simulink model "HANcoder_E407_TTA_Chris"  (R2022b)
settings: Solver=FixedStepDiscrete  StartTime=0.0  StopTime=1  FixedStep=0.01  RelTol=1e-3
PreLoadFcn:
  | librarySetup
  | eval([bdroot,'_startup']) %Calling [modelName]_startup.m
values from neighbouring files (symbols this model uses):
  ClockOn = Simulink.Parameter    [HANcoder_E407_TTA_Chris_startup.m]    (also in HANcoder_E407_TTA_CombineModel_Membership_2022a_startup.m; HANcoder_E407_TTA_CombineModel_Membership_startup.m; HANcoder_E407_TTA_CombineModel_V2_startup.m; HANcoder_E407_TTA_CombineModel_startup.m)
  frequency_IRQ = 1000    [HANcoder_E407_TTA_Chris_startup.m]    (also in HANcoder_E407_TTA_CombineModel_Membership_2022a_startup.m; HANcoder_E407_TTA_CombineModel_Membership_startup.m; HANcoder_E407_TTA_CombineModel_V2_startup.m; HANcoder_E407_TTA_CombineModel_startup.m)
  idA = 4    [HANcoder_E407_TTA_Chris_startup.m]    (also in HANcoder_E407_TTA_CombineModel_Membership_2022a_startup.m; HANcoder_E407_TTA_CombineModel_Membership_startup.m; HANcoder_E407_TTA_CombineModel_V2_startup.m; HANcoder_E407_TTA_CombineModel_startup.m)
  idB = 6    [HANcoder_E407_TTA_Chris_startup.m]    (also in HANcoder_E407_TTA_CombineModel_Membership_2022a_startup.m; HANcoder_E407_TTA_CombineModel_Membership_startup.m; HANcoder_E407_TTA_CombineModel_V2_startup.m; HANcoder_E407_TTA_CombineModel_startup.m)
  matrixRows = Simulink.Parameter    [HANcoder_E407_TTA_Chris_startup.m]    (also in HANcoder_E407_TTA_CombineModel_Membership_2022a_startup.m; HANcoder_E407_TTA_CombineModel_Membership_startup.m; HANcoder_E407_TTA_CombineModel_V2_startup.m; HANcoder_E407_TTA_CombineModel_startup.m)
  MMBS1_ID = Simulink.Parameter    [HANcoder_E407_TTA_Chris_startup.m]    (also in HANcoder_E407_TTA_CombineModel_Membership_2022a_startup.m; HANcoder_E407_TTA_CombineModel_Membership_startup.m; HANcoder_E407_TTA_CombineModel_V2_startup.m; HANcoder_E407_TTA_CombineModel_startup.m)
  slotTime = Simulink.Parameter    [HANcoder_E407_TTA_Chris_startup.m]    (also in HANcoder_E407_TTA_CombineModel_Membership_2022a_startup.m; HANcoder_E407_TTA_CombineModel_Membership_startup.m; HANcoder_E407_TTA_CombineModel_V2_startup.m; HANcoder_E407_TTA_CombineModel_startup.m)
  SSTM1_ID = Simulink.Parameter    [HANcoder_E407_TTA_Chris_startup.m]    (also in HANcoder_E407_TTA_CombineModel_Membership_2022a_startup.m; HANcoder_E407_TTA_CombineModel_Membership_startup.m; HANcoder_E407_TTA_CombineModel_V2_startup.m; HANcoder_E407_TTA_CombineModel_startup.m)
  SYNC1_ID = Simulink.Parameter    [HANcoder_E407_TTA_Chris_startup.m]    (also in HANcoder_E407_TTA_CombineModel_Membership_2022a_startup.m; HANcoder_E407_TTA_CombineModel_Membership_startup.m; HANcoder_E407_TTA_CombineModel_V2_startup.m; HANcoder_E407_TTA_CombineModel_startup.m)
  TRCK1_ID1 = Simulink.Parameter    [HANcoder_E407_TTA_Chris_startup.m]    (also in HANcoder_E407_TTA_CombineModel_Membership_2022a_startup.m; HANcoder_E407_TTA_CombineModel_Membership_startup.m; HANcoder_E407_TTA_CombineModel_V2_startup.m; HANcoder_E407_TTA_CombineModel_startup.m)
  TRCK1_ID2 = Simulink.Parameter    [HANcoder_E407_TTA_Chris_startup.m]    (also in HANcoder_E407_TTA_CombineModel_Membership_2022a_startup.m; HANcoder_E407_TTA_CombineModel_Membership_startup.m; HANcoder_E407_TTA_CombineModel_V2_startup.m; HANcoder_E407_TTA_CombineModel_startup.m)
  TRCK1_ID3 = Simulink.Parameter    [HANcoder_E407_TTA_Chris_startup.m]    (also in HANcoder_E407_TTA_CombineModel_Membership_2022a_startup.m; HANcoder_E407_TTA_CombineModel_Membership_startup.m; HANcoder_E407_TTA_CombineModel_V2_startup.m; HANcoder_E407_TTA_CombineModel_startup.m)
  TRLS1_ID4 = Simulink.Parameter    [HANcoder_E407_TTA_Chris_startup.m]    (also in HANcoder_E407_TTA_CombineModel_Membership_2022a_startup.m; HANcoder_E407_TTA_CombineModel_Membership_startup.m; HANcoder_E407_TTA_CombineModel_V2_startup.m; HANcoder_E407_TTA_CombineModel_startup.m)
  TRLS1_ID5 = Simulink.Parameter    [HANcoder_E407_TTA_Chris_startup.m]    (also in HANcoder_E407_TTA_CombineModel_Membership_2022a_startup.m; HANcoder_E407_TTA_CombineModel_Membership_startup.m; HANcoder_E407_TTA_CombineModel_V2_startup.m; HANcoder_E407_TTA_CombineModel_startup.m)
libraries: HANcoder_STM32_Target x14, simulink_extras x1
(part 1 of 3)
settings Model: Creator=Jason van Kolfschoten  LastModifiedBy=Admin.cvanderspek
settings SolverCC: AlgebraicLoopSolver=TrustRegion  PositivePriorityOrder=on
settings DataIOCC: LimitDataPoints=on  SaveFormat=Array  SignalLoggingSaveFormat=ModelDataLogs  SaveOutput=off  SignalLogging=off  DSMLogging=off  SaveTime=off  ReturnWorkspaceOutputs=off
settings OptimizationCC: BlockReduction=off  DefaultParameterBehavior=Inlined  DefaultUnderspecifiedDataType=single  InlineInvariantSignals=on  ExpressionDepthLimit=2147483647  StateBitsets=on  DataBitsets=on  ZeroExternalMemoryAtStartup=off  ZeroInternalMemoryAtStartup=off  InitFltsAndDblsToZero=on  NoFixptDivByZeroProtection=on  EfficientFloat2IntCast=on  LifeSpan=inf  EfficientTunableParamExpr=on
settings DebuggingCC: SaveWithDisabledLinksMsg=none  SaveWithParameterizedLinksMsg=none  CheckSSInitialOutputMsg=off  UnderspecifiedInitializationDetection=Classic  MergeDetectMultiDrivingBlocksExec=none  SignalResolutionControl=TryResolveAll  SolverPrmCheckMsg=warning  InheritedTsInSrcMsg=none  MultiTaskDSMMsg=warning  MultiTaskCondExecSysMsg=none  ParameterPrecisionLossMsg=none  FcnCallInpInsideContextMsg=warning  UnconnectedInputMsg=warning  UnconnectedOutputMsg=warning  UnconnectedLineMsg=warning  StateNameClashWarn=warning  SFUnexpectedBacktrackingDiag=warning  SFNoUnconditionalDefaultTransitionDiag=warning  SFExecutionAtInitializationDiag=none  SFMachineParentedDataDiag=warning  ArithmeticOperatorsInVariantConditions=warning
settings HardwareCC: ProdBitPerPointer=32  ProdBitPerSizeT=32  ProdBitPerPtrDiffT=32  ProdLargestAtomicInteger=Long  ProdLargestAtomicFloat=Double  ProdWordSize=32  ProdHWDeviceType=ARM Compatible->ARM Cortex  TargetEndianess=LittleEndian  TargetHWDeviceType=Infineon->TriCore
settings ModelReferenceCC: PropagateSignalLabelsOutOfModel=off
settings SFSimCC: SimUseLocalCustomCode=off  MATLABDynamicMemAlloc=off  CustomCodeUndefinedFunction=UseInterfaceOnly
settings RTWCC: Description=Real-Time Workshop Embedded Coder (no auto configuration)  SystemTargetFile=ert.tlc  MakeCommand=make_rtw SHELL= HANcoder_PORTABLE=1 HANcoder_BOOTLOADER=1  TemplateMakefile=STM32_E407_gcc.tmf  RTWUseLocalCustomCode=off
settings CodeAppCC: ForceParamTrailComments=on  IgnoreCustomStorageClasses=off  SimulinkDataObjDesc=on  CustomSymbolStrGlobalVar=rt$N$M  CustomSymbolStrType=$N$M  CustomSymbolStrFcn=$N$M$F  CustomSymbolStrMacro=$N$M  InsertBlockDesc=on  StateflowObjectComments=on  InternalIdentifier=Classic
settings ERTTargetCC: TargetFcnLib=ansi_tfl_tmw.mat  MultiwordLength=2048  IncludeMdlTerminateFcn=off  SuppressErrorStatus=on  SupportNonFinite=off  GenerateASAP2=on  InlinedParameterPlacement=NonHierarchical  ERTCustomFileTemplate=example_file_process.tlc  ConvertIfToSwitch=off  SuppressUnreachableDefaultCases=off
settings ConfigComp: CovMetricSettings=dw  CovSaveCumulativeToWorkspaceVar=on  CovSaveSingleToWorkspaceVar=on  CovExternalEMLEnable=off  CovSFcnEnable=off  DVMaxProcessTime=600  DVAutomaticStubbing=off  DVModelCoverageObjectives=MCDC  DVMaxTestCaseSteps=500  DVTestSuiteOptimization=CombinedObjectives  DVDetectActiveLogic=on  DVSaveHarnessModel=on  DVHarnessSource=Signal Editor

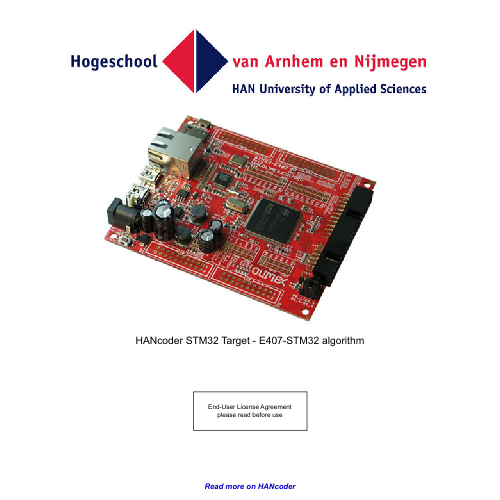
[thumbnail: Simulink's stored preview of the top-level diagram]
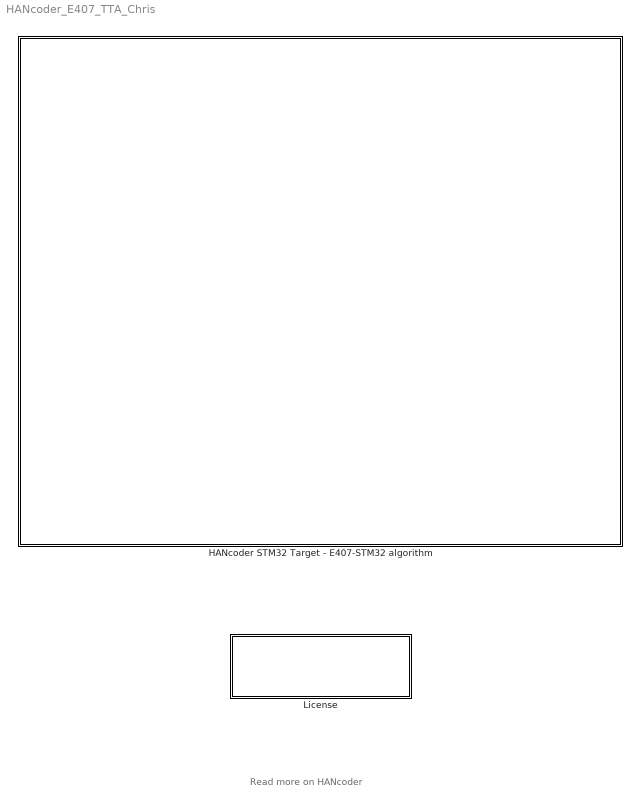
== system HANcoder_E407_TTA_Chris ==
  note: Read more on HANcoder
  HANcoder STM32 Target - E407-STM32 algorithm : Subsystem  mask(TopLevelSubsystem){}
      settings: CopyFcn=HANcoderChecks('Copy');  NameChangeFcn=HANcoderChecks('NameChangeE407');  MoveFcn=HANcoderChecks('MoveE407');
      mask Display: image(imread('STM32_E407_HAN.jpg'))
  License : Subsystem  mask(License){}
      settings: NameChangeFcn=HANcoderChecks('NameChangeLicenseBlock');  OpenFcn=winopen('License.pdf')  MoveFcn=HANcoderChecks('MoveLicenseBlock');
      mask Display: disp(['End-User License Agreement\n','please read before use']);

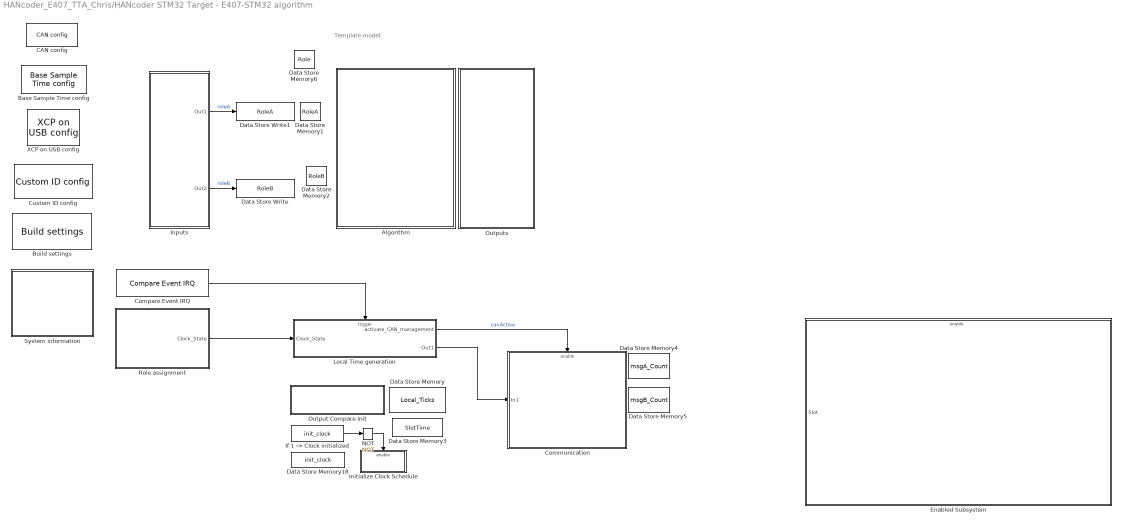
== system HANcoder_E407_TTA_Chris/HANcoder STM32 Target - E407-STM32 algorithm ==
  note: Template model
  Algorithm : Subsystem
  Base Sample Time config : HANcoder_STM32_Target/STM32-E407/System Config/Base Sample Time config  Tag=HANcoder_TARGET_STM32_E407  Description=HANcoder Target STM32-E407 blockset version 1.0  baseSampleTime=10  extraStack=100
  Build settings : HANcoder_STM32_Target/STM32-E407/System Config/Build settings  Tag=HANcoder_TARGET_STM32_E407  AutoASAP2add=on  AutoFlash=USB
  CAN config : HANcoder_STM32_Target/STM32-E407/System Config/CAN config  Tag=HANcoder_TARGET_STM32_E407  txBufSize=64  evBufSize=8  canBus1=on  baudRate1=250  rxMask1=hex2dec('00000000')  rxCode1=hex2dec('00000000')  rxMode1=Receive only 11-bit message identifiers  canBus2=off  baudRate2=250  rxMask2=hex2dec('00000000')  rxCode2=hex2dec('00000000')  rxMode2=Receive only 11-bit message identifiers
  Communication : Subsystem
  Compare Event IRQ : HANcoder_STM32_Target/STM32-E407/Timer Outputs/Compare Event IRQ  Tag=HANcoder_TARGET_STM32_E407  Priority=20  pin=TIM4 - CON PD - 15 - 5V Tolerant
  Custom ID config : HANcoder_STM32_Target/STM32-E407/System Config/Custom ID config  Tag=HANcoder_TARGET_STM32_E407  softID=softwareID  softNUM=1
  Data Store Memory : DataStoreMemory  DataStoreName=Local_Ticks  WriteAfterWriteMsg=warning  ShowAdditionalParam=off  OutDataTypeStr=uint16
  Data Store Memory1 : DataStoreMemory  DataStoreName=RoleA  WriteAfterWriteMsg=warning  ShowAdditionalParam=off  OutDataTypeStr=boolean
  Data Store Memory18 : DataStoreMemory  Priority=1  DataStoreName=init_clock  ReadBeforeWriteMsg=warning  WriteAfterWriteMsg=warning  WriteAfterReadMsg=warning  ShowAdditionalParam=off
  Data Store Memory2 : DataStoreMemory  DataStoreName=RoleB  WriteAfterWriteMsg=warning  ShowAdditionalParam=off  OutDataTypeStr=boolean
  Data Store Memory3 : DataStoreMemory  DataStoreName=SlotTime  WriteAfterWriteMsg=warning  ShowAdditionalParam=off  OutDataTypeStr=uint8
  Data Store Memory4 : DataStoreMemory  DataStoreName=msgA_Count  WriteAfterWriteMsg=warning  ShowAdditionalParam=off  OutDataTypeStr=uint8
  Data Store Memory5 : DataStoreMemory  DataStoreName=msgB_Count  WriteAfterWriteMsg=warning  ShowAdditionalParam=off  OutDataTypeStr=uint8
  Data Store Memory6 : DataStoreMemory  DataStoreName=Role  WriteAfterWriteMsg=warning  ShowAdditionalParam=off  OutDataTypeStr=boolean
  Data Store Write : DataStoreWrite  DataStoreName=RoleB  IndexOptions=Index vector (dialog)  Indices=1  OutputSizes=1
  Data Store Write1 : DataStoreWrite  DataStoreName=RoleA  IndexOptions=Index vector (dialog)  Indices=1  OutputSizes=1
  Enabled Subsystem : Subsystem  TreatAsAtomicUnit=on
  "If 1 -> Clock initialized " : DataStoreRead  Priority=2  DataStoreName=init_clock  IndexOptions=Index vector (dialog)  Indices=1  OutputSizes=1
  Initialize Clock Schedule : Subsystem  Priority=4  TreatAsAtomicUnit=on
  Inputs : Subsystem
  Local Time generation : Subsystem  TreatAsAtomicUnit=on
  NOT : Logic  Priority=3  Operator=NOT  IconShape=distinctive  AllPortsSameDT=off  OutDataTypeStr=boolean
  Output Compare Init : Subsystem  Tag=HANcoder_TARGET_STM32_E407  AncestorBlock=HANcoder_STM32_Target/STM32-E407/Timer Outputs/Output Compare Init  mask(Output Compare Init){moduleID=TIM4 - CON PD - 15 & 16 &n/a & n/a, frequency=1000000, enableIRQoutput=off}
      mask prompts: moduleID "Timer module"; frequency "Frequency (free running counter) [Hz]"; enableIRQoutput "Enable IRQ output"
      mask help:
      | Function
      | ========
      | Initializes the timer module to allow output compare functionality on the
      | module's channels.
      |
      | Parameters
      | ==========
      | Timer Module:
      |   Selects the timer module.
      |
      | Frequency:
      |   Frequency at which the 16-bit free running counter counts.
      |
      | Enable IRQ output
      |   Controls whether or not the IRQ output is available.
      |
      | Outport
      | =======
      | IRQ
      |   Allows connection of a function call subsystem for the free running
      |   counter overflow event.
      mask init:
      | moduleIDInfoStr = sfcn_timeout_init_mcb(2, moduleID, frequency, enableIRQoutput);
      settings: LibrarySourceBlock=HANcoder_STM32_Target/STM32-E407/Timer Outputs/Output Compare Init  CopyFcn=sfcn_timeout_init_chk();  MoveFcn=drawLogos
      mask Help: web('sfcn_timeout_init.html');
      mask TypeOptions moduleID: TIM1 - CON PE - 12 & 14 & 16 & 17 | TIM2 - CON4 - D13 & n/a & n/a & n/a | TIM3 - CON4 - D12 & D11 & n/a & n/a | TIM4 - CON PD - 15 & 16 &n/a & n/a | TIM8 - UEXT - 3 & 4 & n/a & n/a | TIM9 - CON3 - D4 & D5 or PE - 8 & 9 | TIM10 - CON2 - A1 or CON PF - 9 | TIM11 - CON2 - A2 or CON PF - 10 | TIM13 - CON2 - A3 or CON PF - 11 | TIM14 - CON2 - A4 or CON PF - 12
      mask Callback moduleID: sfcn_timeout_init_chk();
      mask Display: fprintf('Output Compare Init\n%s', moduleIDInfoStr);patch([135 141 141],[8 14 2],[1 0 0]);patch([143 143 149],[14 2 8],[0 0 0.35]);
  Outputs : Subsystem
  Role assignment : Subsystem
  System information : Subsystem
  XCP on USB config : HANcoder_STM32_Target/STM32-E407/System Config/XCP on USB config  Tag=HANcoder_TARGET_STM32_E407
  wires:
  Compare Event IRQ/1 -> Local Time generation/Trigger
  Inputs/1(Out1) -> Data Store Write1/1  "roleA"
  Inputs/2(Out2) -> Data Store Write/1  "roleB"
  NOT/1 -> Initialize Clock Schedule/Enable
  "If 1 -> Clock initialized "/1 -> NOT/1
  Local Time generation/1(activate_CAN_management) -> Communication/Enable  "canActive"
  Local Time generation/2(Out1) -> Communication/1(In1)
  Role assignment/1(Clock_State) -> Local Time generation/1(Clock_State)

== system HANcoder_E407_TTA_Chris/License ==

== system HANcoder_E407_TTA_Chris/HANcoder STM32 Target - E407-STM32 algorithm/Algorithm ==
  note: Here the algorithm can be placed. No hardware dependent blocks should be used here.

== system HANcoder_E407_TTA_Chris/HANcoder STM32 Target - E407-STM32 algorithm/Communication ==
  In1 : Inport
  Enable : EnablePort
  MatrixScheduler : Subsystem
  Role A Rx : Subsystem
  Role A Tx : Subsystem
  Role B Rx : Subsystem
  Role B Tx : Subsystem
  wires:
  MatrixScheduler/1(Out1) -> Role A Tx/Trigger
  MatrixScheduler/2(Out2) -> Role A Rx/Enable
  In1/1 -> MatrixScheduler/1(In1)
  MatrixScheduler/3(Out3) -> Role B Rx/Enable
  MatrixScheduler/4(Out4) -> Role B Tx/Trigger

== system HANcoder_E407_TTA_Chris/HANcoder STM32 Target - E407-STM32 algorithm/Enabled Subsystem ==
  Slot : Inport
  Enable : EnablePort
  Constant4 : Constant  Value=5
  Equal4 : RelationalOperator  Operator===  OutDataTypeStr=boolean  RndMeth=Simplest  InputSameDT=off
  Trailer 2 : Subsystem  TreatAsAtomicUnit=on
  Truck 1 : Subsystem  Description=Truck 1  TreatAsAtomicUnit=on
  wires:
  Equal4/1 -> Trailer 2/Enable
  Constant4/1 -> Equal4/2
  Slot/1 -> Truck 1/1(Slot)

== system HANcoder_E407_TTA_Chris/HANcoder STM32 Target - E407-STM32 algorithm/Initialize Clock Schedule ==
  Enable : EnablePort
  Constant : Constant  OutDataTypeStr=uint16
  Constant1 : Constant  Value=3  OutDataTypeStr=uint8
  Constant2 : Constant
  Data Store Write : DataStoreWrite  DataStoreName=init_clock  IndexOptions=Index vector (dialog)  Indices=1  OutputSizes=1
  Schedule Compare Event : HANcoder_STM32_Target/STM32-E407/Timer Outputs/Schedule Compare Event  Tag=HANcoder_TARGET_STM32_E407  pin=TIM4 - CON PD - 15 - 5V Tolerant  tsamp=-1
  wires:
  Constant/1 -> Schedule Compare Event/1
  Constant1/1 -> Schedule Compare Event/2
  Constant2/1 -> Data Store Write/1

== system HANcoder_E407_TTA_Chris/HANcoder STM32 Target - E407-STM32 algorithm/Inputs ==
  note: The inputs and outputs are kept in a separate subsystem, this way the algorithm can easily be transferred to different hardware
  Cast : DataTypeConversion  OutDataTypeStr=boolean  SaturateOnIntegerOverflow=off  RndMeth=Floor
  Cast1 : DataTypeConversion  OutDataTypeStr=boolean  SaturateOnIntegerOverflow=off  RndMeth=Floor
  Digital Input : HANcoder_STM32_Target/STM32-E407/Digital Inputs/Digital Input  Tag=HANcoder_TARGET_STM32_E407  pinID=CON3 - D2 - 5V Tolerant  config=Pulldown  tsamp=-1
  Digital Input1 : HANcoder_STM32_Target/STM32-E407/Digital Inputs/Digital Input  Tag=HANcoder_TARGET_STM32_E407  pinID=CON3 - D3 - 5V Tolerant  config=Pulldown  tsamp=-1
  Out1 : Outport
  Out2 : Outport  Port=2
  wires:
  Digital Input1/1 -> Cast/1
  Digital Input/1 -> Cast1/1
  Cast1/1 -> Out2/1
  Cast/1 -> Out1/1

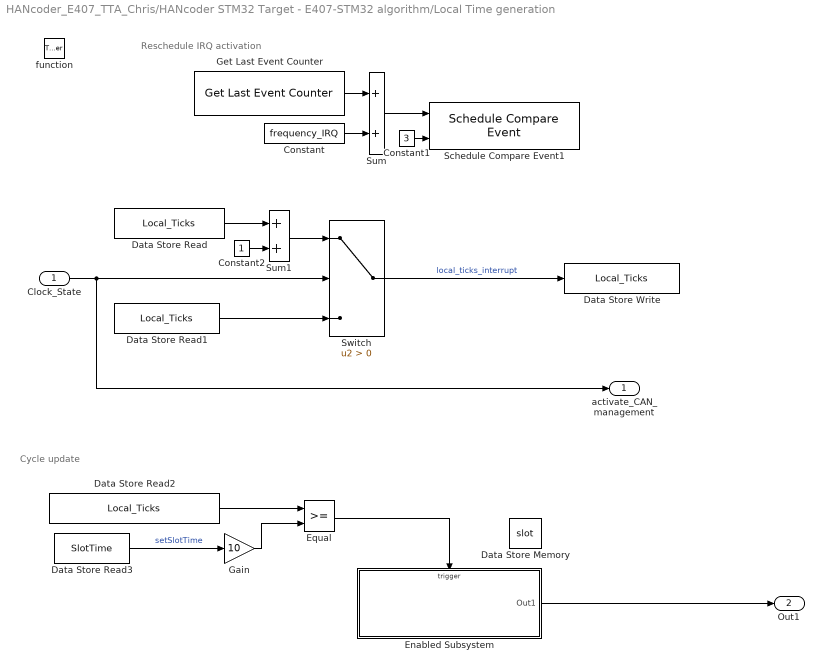
== system HANcoder_E407_TTA_Chris/HANcoder STM32 Target - E407-STM32 algorithm/Local Time generation ==
  note: Reschedule IRQ activation
  note: Cycle update
  Clock_State : Inport
  function : TriggerPort  TriggerType=function-call  VariantControl=Variant
  Constant : Constant  Value=frequency_IRQ  OutDataTypeStr=uint16
  Constant1 : Constant  Value=3  OutDataTypeStr=uint8
  Constant2 : Constant  OutDataTypeStr=uint16
  Data Store Memory : DataStoreMemory  DataStoreName=slot  WriteAfterWriteMsg=warning  ShowAdditionalParam=off  OutDataTypeStr=uint8
  Data Store Read : DataStoreRead  DataStoreName=Local_Ticks  IndexOptions=Index vector (dialog)  Indices=1  OutputSizes=1
  Data Store Read1 : DataStoreRead  DataStoreName=Local_Ticks  IndexOptions=Index vector (dialog)  Indices=1  OutputSizes=1
  Data Store Read2 : DataStoreRead  DataStoreName=Local_Ticks  IndexOptions=Index vector (dialog)  Indices=1  OutputSizes=1
  Data Store Read3 : DataStoreRead  DataStoreName=SlotTime  IndexOptions=Index vector (dialog)  Indices=1  OutputSizes=1
  Data Store Write : DataStoreWrite  DataStoreName=Local_Ticks  IndexOptions=Index vector (dialog)  Indices=1  OutputSizes=1
  Enabled Subsystem : Subsystem  TreatAsAtomicUnit=on
  Equal : RelationalOperator  OutDataTypeStr=boolean  RndMeth=Simplest  InputSameDT=off
  Gain : Gain  Gain=10  OutDataTypeStr=uint16
  Get Last Event Counter : HANcoder_STM32_Target/STM32-E407/Timer Outputs/Get Last Event Counter  Tag=HANcoder_TARGET_STM32_E407  pin=TIM4 - CON PD - 15 - 5V Tolerant  tsamp=-1
  Schedule Compare Event1 : HANcoder_STM32_Target/STM32-E407/Timer Outputs/Schedule Compare Event  Tag=HANcoder_TARGET_STM32_E407  pin=TIM4 - CON PD - 15 - 5V Tolerant  tsamp=-1
  Sum : Sum
  Sum1 : Sum
  Switch : Switch  Criteria=u2 > Threshold  SaturateOnIntegerOverflow=off  InputSameDT=off
  activate_CAN_management : Outport  VectorParamsAs1DForOutWhenUnconnected=off
  Out1 : Outport  Port=2
  wires:
  Get Last Event Counter/1 -> Sum/1
  Constant/1 -> Sum/2
  Sum/1 -> Schedule Compare Event1/1
  Constant1/1 -> Schedule Compare Event1/2
  Data Store Read1/1 -> Switch/3
  Data Store Read/1 -> Sum1/1
  Constant2/1 -> Sum1/2
  Switch/1 -> Data Store Write/1  "local_ticks_interrupt"
  Sum1/1 -> Switch/1
  Clock_State/1 -> activate_CAN_management/1, Switch/2
  Data Store Read2/1 -> Equal/1
  Enabled Subsystem/1(Out1) -> Out1/1
  Equal/1 -> Enabled Subsystem/Trigger
  Data Store Read3/1 -> Gain/1  "setSlotTime"
  Gain/1 -> Equal/2

== system HANcoder_E407_TTA_Chris/HANcoder STM32 Target - E407-STM32 algorithm/Output Compare Init ==
  S-Function : S-Function  FunctionName=sfcn_timeout_init  SFunctionDeploymentMode=off  EnableBusSupport=off
  Term1 : Terminator
  wires:
  S-Function/1 -> Term1/1

== system HANcoder_E407_TTA_Chris/HANcoder STM32 Target - E407-STM32 algorithm/Outputs ==
  note: The inputs and outputs are kept in a separate subsystem, this way the algorithm can easily be transferred to different hardware

== system HANcoder_E407_TTA_Chris/HANcoder STM32 Target - E407-STM32 algorithm/Role assignment ==
  AND : Logic  IconShape=distinctive  AllPortsSameDT=off  OutDataTypeStr=boolean
  Constant : Constant  Value=ClockOn
  Data Store Read : DataStoreRead  DataStoreName=RoleA  IndexOptions=Index vector (dialog)  Indices=1  OutputSizes=1
  Data Store Read1 : DataStoreRead  DataStoreName=RoleB  IndexOptions=Index vector (dialog)  Indices=1  OutputSizes=1
  OR : Logic  Operator=OR  IconShape=distinctive  AllPortsSameDT=off  OutDataTypeStr=boolean
  Subsystem : Subsystem
  Subsystem1 : Subsystem
  Clock_State : Outport
  wires:
  Data Store Read1/1 -> Subsystem1/Enable
  Constant/1 -> AND/1
  OR/1 -> Clock_State/1
  Data Store Read/1 -> AND/2
  Subsystem1/1(Out1) -> OR/2
  AND/1 -> OR/1, Subsystem/Trigger

== system HANcoder_E407_TTA_Chris/HANcoder STM32 Target - E407-STM32 algorithm/System information ==
  note: These blocks check the free memory: stack and heap and the CPU load,
      | this way you can see whether your software demands too much of the microcontroller
  Get CPU load : HANcoder_STM32_Target/STM32-E407/System Management/Get CPU load  Tag=HANcoder_TARGET_STM32_E407  mode=Current CPU load  tsamp=-1
  Get free Heap : HANcoder_STM32_Target/STM32-E407/System Management/Get free Heap  Tag=HANcoder_TARGET_STM32_E407  tsamp=-1
  Get free Stack : HANcoder_STM32_Target/STM32-E407/System Management/Get free Stack  Tag=HANcoder_TARGET_STM32_E407  taskIdx=Application Control Task  tsamp=-1
  Terminator : Terminator
  Terminator1 : Terminator
  Terminator2 : Terminator
  wires:
  Get CPU load/1 -> Terminator1/1  "SI_CPUload"
  Get free Stack/1 -> Terminator/1  "SI_FreeStack"
  Get free Heap/1 -> Terminator2/1  "SI_FreeHeap"

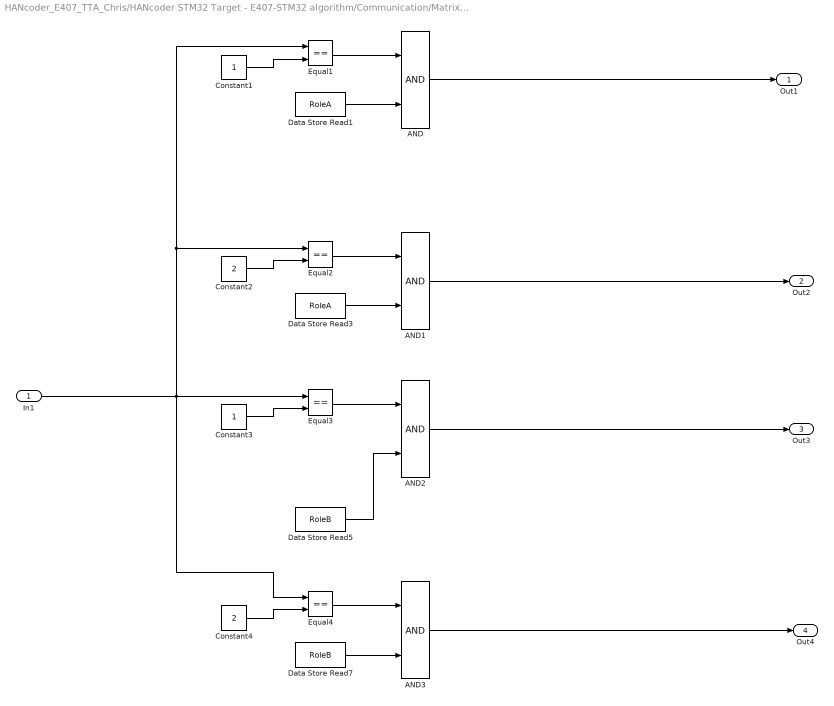
== system HANcoder_E407_TTA_Chris/HANcoder STM32 Target - E407-STM32 algorithm/Communication/MatrixScheduler ==
  In1 : Inport
  AND{,1..3} (4 alike) : Logic  IconShape=distinctive  AllPortsSameDT=off  OutDataTypeStr=boolean
  Constant1 : Constant
  Constant2 : Constant  Value=2
  Constant3 : Constant
  Constant4 : Constant  Value=2
  Data Store Read1 : DataStoreRead  DataStoreName=RoleA  IndexOptions=Index vector (dialog)  Indices=1  OutputSizes=1
  Data Store Read3 : DataStoreRead  DataStoreName=RoleA  IndexOptions=Index vector (dialog)  Indices=1  OutputSizes=1
  Data Store Read5 : DataStoreRead  DataStoreName=RoleB  IndexOptions=Index vector (dialog)  Indices=1  OutputSizes=1
  Data Store Read7 : DataStoreRead  DataStoreName=RoleB  IndexOptions=Index vector (dialog)  Indices=1  OutputSizes=1
  Equal{1..4} (4 alike) : RelationalOperator  Operator===  OutDataTypeStr=boolean  RndMeth=Simplest  InputSameDT=off
  Out1 : Outport
  Out2 : Outport  Port=2
  Out3 : Outport  Port=3
  Out4 : Outport  Port=4
  wires:
  Equal1/1 -> AND/1
  AND2/1 -> Out3/1
  Constant3/1 -> Equal3/2
  Data Store Read3/1 -> AND1/2
  Equal4/1 -> AND3/1
  Data Store Read5/1 -> AND2/2
  Equal3/1 -> AND2/1
  Equal2/1 -> AND1/1
  Constant2/1 -> Equal2/2
  Constant4/1 -> Equal4/2
  Data Store Read1/1 -> AND/2
  Constant1/1 -> Equal1/2
  In1/1 -> Equal4/1, Equal1/1, Equal2/1, Equal3/1
  Data Store Read7/1 -> AND3/2
  AND1/1 -> Out2/1
  AND/1 -> Out1/1
  AND3/1 -> Out4/1

== system HANcoder_E407_TTA_Chris/HANcoder STM32 Target - E407-STM32 algorithm/Communication/Role A Rx ==
  Enable : EnablePort
  CAN receive1 : Subsystem  Tag=HANcoder_TARGET_STM32_E407  AncestorBlock=HANcoder_STM32_Target/STM32-E407/CAN/CAN/CAN receive  mask(CAN receive){canBus=CAN 1, outputNumber=1, dataType=uint8, byteOrder=off, tsamp=-1}
      mask prompts: canBus "CAN channel"; outputNumber "Output ports"; dataType "Output datatype"; byteOrder "Byte order: Checked = MSB first, unchecked = LSB first."; tsamp "Sample time"
      mask help:
      | Function
      | ==========
      | Receive the newest message from the specified CAN channel.
      |
      | Parameters
      | ==========
      | CAN channel:             The CAN channel to send the message on.
      | Output ports:             The amount of output ports
      | Output datatype:       The datatype of the output ports
      | Byte order:                 Select MSB or LSB first
      | Sample time:              -1 or divisible by base sample time [seconds]
      |
      | Input
      | ==========
      | Port 1:                       CAN ID(uint32) in hexadecimal ie: hex2dec('0a')
      |
      | Output
      | ==========
      | Port 1:                       Checks for new message(int8)
      | Port 2..9                     Message data
      mask init:
      | sfcn_can_receive_mcb(canBus, outputNumber, dataType, byteOrder)
      settings: LibrarySourceBlock=HANcoder_STM32_Target/STM32-E407/CAN/CAN/CAN receive  MoveFcn=drawLogos
      mask Help: web('sfcn_can_receive.html');
      mask TypeOptions canBus: CAN 1 | CAN 2
      mask TypeOptions dataType: int8 | uint8 | int16 | uint16 | int32 | uint32 | boolean
      mask Display:
      | fprintf('Receive on\nCAN %x', canBus);
      | port_label('output', 1, 'new');
      | port_label('input', 1, 'ID');patch([210 216 216],[8 14 2],[1 0 0]);patch([218 218 224],[14 2 8],[0 0 0.35]);
  Constant : Constant  Value=idB  OutDataTypeStr=uint32
  Terminator : Terminator
  Terminator1 : Terminator
  wires:
  Constant/1 -> CAN receive1/1(In1)
  CAN receive1/1(Out1) -> Terminator1/1
  CAN receive1/2(Out2) -> Terminator/1  "dataArx"

== system HANcoder_E407_TTA_Chris/HANcoder STM32 Target - E407-STM32 algorithm/Communication/Role A Tx ==
  Trigger : TriggerPort  VariantControl=(inherit)  PortDimensions=1
  Add : Sum
  CAN send1 : Subsystem  Tag=HANcoder_TARGET_STM32_E407  AncestorBlock=HANcoder_STM32_Target/STM32-E407/CAN/CAN/CAN send  mask(CAN send){canBus=CAN 1, frameType=Standard (11 bit), inputNumber=1, dataType=uint8, byteOrder=on, tsamp=-1}
      mask prompts: canBus "CAN channel"; frameType "Identifier type"; inputNumber "Input ports"; dataType "Input datatype"; byteOrder "Byte order: Checked = MSB first, unchecked = LSB first."; tsamp "Sample time"
      mask help:
      | Function
      | ==========
      | Send a message on the CAN channel.
      |
      | Parameters
      | ==========
      | CAN channel:           The CAN channel to send the message on.
      | Identifier type:         normal or extended ID's
      | Input ports:              The amount of input ports
      | Input datatype:        The datatype of the input ports
      | Byte order:               Select MSB or LSB first
      | Sample time:            -1 or divisible by base sample time [seconds]
      |
      | Input
      | ==========
      | Port 1:                   CAN ID(uint32) in hexadecimal ie: hex2dec('0a')
      | Port 2..9                CAN message data
      mask init:
      | sfcn_can_send_mcb(canBus, frameType, inputNumber, dataType, byteOrder)
      settings: LibrarySourceBlock=HANcoder_STM32_Target/STM32-E407/CAN/CAN/CAN send  MoveFcn=drawLogos
      mask Help: web('sfcn_can_send.html');
      mask TypeOptions canBus: CAN 1 | CAN 2
      mask TypeOptions frameType: Standard (11 bit) | Extended (29 bit)
      mask TypeOptions dataType: int8 | uint8 | int16 | uint16 | int32 | uint32 | boolean
      mask Display:
      | fprintf('Send on\nCAN %x', canBus);
      | port_label('input', 1, 'ID');patch([200 206 206],[8 14 2],[1 0 0]);patch([208 208 214],[14 2 8],[0 0 0.35]);
  Constant : Constant  Value=idA  OutDataTypeStr=uint32
  Constant1 : Constant  OutDataTypeStr=uint8
  Data Store Read : DataStoreRead  DataStoreName=msgA_Count  IndexOptions=Index vector (dialog)  Indices=1  OutputSizes=1
  Data Store Write : DataStoreWrite  DataStoreName=msgA_Count  IndexOptions=Index vector (dialog)  Indices=1  OutputSizes=1
  wires:
  Constant/1 -> CAN send1/1(In1)
  Add/1 -> CAN send1/2(In2), Data Store Write/1  "dataAtx"
  Data Store Read/1 -> Add/1
  Constant1/1 -> Add/2

== system HANcoder_E407_TTA_Chris/HANcoder STM32 Target - E407-STM32 algorithm/Communication/Role B Rx ==
  Enable : EnablePort
  CAN receive1 : Subsystem  Tag=HANcoder_TARGET_STM32_E407  AncestorBlock=HANcoder_STM32_Target/STM32-E407/CAN/CAN/CAN receive  mask(CAN receive){canBus=CAN 1, outputNumber=1, dataType=uint8, byteOrder=off, tsamp=-1}
      mask prompts: canBus "CAN channel"; outputNumber "Output ports"; dataType "Output datatype"; byteOrder "Byte order: Checked = MSB first, unchecked = LSB first."; tsamp "Sample time"
      mask help:
      | Function
      | ==========
      | Receive the newest message from the specified CAN channel.
      |
      | Parameters
      | ==========
      | CAN channel:             The CAN channel to send the message on.
      | Output ports:             The amount of output ports
      | Output datatype:       The datatype of the output ports
      | Byte order:                 Select MSB or LSB first
      | Sample time:              -1 or divisible by base sample time [seconds]
      |
      | Input
      | ==========
      | Port 1:                       CAN ID(uint32) in hexadecimal ie: hex2dec('0a')
      |
      | Output
      | ==========
      | Port 1:                       Checks for new message(int8)
      | Port 2..9                     Message data
      mask init:
      | sfcn_can_receive_mcb(canBus, outputNumber, dataType, byteOrder)
      settings: LibrarySourceBlock=HANcoder_STM32_Target/STM32-E407/CAN/CAN/CAN receive  MoveFcn=drawLogos
      mask Help: web('sfcn_can_receive.html');
      mask TypeOptions canBus: CAN 1 | CAN 2
      mask TypeOptions dataType: int8 | uint8 | int16 | uint16 | int32 | uint32 | boolean
      mask Display:
      | fprintf('Receive on\nCAN %x', canBus);
      | port_label('output', 1, 'new');
      | port_label('input', 1, 'ID');patch([210 216 216],[8 14 2],[1 0 0]);patch([218 218 224],[14 2 8],[0 0 0.35]);
  Constant : Constant  Value=idA  OutDataTypeStr=uint32
  Terminator : Terminator
  Terminator1 : Terminator
  wires:
  Constant/1 -> CAN receive1/1(In1)
  CAN receive1/1(Out1) -> Terminator/1
  CAN receive1/2(Out2) -> Terminator1/1  "dataBrx"

== system HANcoder_E407_TTA_Chris/HANcoder STM32 Target - E407-STM32 algorithm/Communication/Role B Tx ==
  Trigger : TriggerPort  VariantControl=(inherit)  PortDimensions=1
  Add : Sum  Inputs=+-  AccumDataTypeStr=uint8
  CAN send1 : Subsystem  Tag=HANcoder_TARGET_STM32_E407  AncestorBlock=HANcoder_STM32_Target/STM32-E407/CAN/CAN/CAN send  mask(CAN send){canBus=CAN 1, frameType=Standard (11 bit), inputNumber=1, dataType=uint8, byteOrder=on, tsamp=-1}
      mask prompts: canBus "CAN channel"; frameType "Identifier type"; inputNumber "Input ports"; dataType "Input datatype"; byteOrder "Byte order: Checked = MSB first, unchecked = LSB first."; tsamp "Sample time"
      mask help:
      | Function
      | ==========
      | Send a message on the CAN channel.
      |
      | Parameters
      | ==========
      | CAN channel:           The CAN channel to send the message on.
      | Identifier type:         normal or extended ID's
      | Input ports:              The amount of input ports
      | Input datatype:        The datatype of the input ports
      | Byte order:               Select MSB or LSB first
      | Sample time:            -1 or divisible by base sample time [seconds]
      |
      | Input
      | ==========
      | Port 1:                   CAN ID(uint32) in hexadecimal ie: hex2dec('0a')
      | Port 2..9                CAN message data
      mask init:
      | sfcn_can_send_mcb(canBus, frameType, inputNumber, dataType, byteOrder)
      settings: LibrarySourceBlock=HANcoder_STM32_Target/STM32-E407/CAN/CAN/CAN send  MoveFcn=drawLogos
      mask Help: web('sfcn_can_send.html');
      mask TypeOptions canBus: CAN 1 | CAN 2
      mask TypeOptions frameType: Standard (11 bit) | Extended (29 bit)
      mask TypeOptions dataType: int8 | uint8 | int16 | uint16 | int32 | uint32 | boolean
      mask Display:
      | fprintf('Send on\nCAN %x', canBus);
      | port_label('input', 1, 'ID');patch([200 206 206],[8 14 2],[1 0 0]);patch([208 208 214],[14 2 8],[0 0 0.35]);
  Constant : Constant  Value=idB  OutDataTypeStr=uint32
  Constant1 : Constant  OutDataTypeStr=uint8
  Data Store Read : DataStoreRead  DataStoreName=msgB_Count  IndexOptions=Index vector (dialog)  Indices=1  OutputSizes=1
  Data Store Write : DataStoreWrite  DataStoreName=msgB_Count  IndexOptions=Index vector (dialog)  Indices=1  OutputSizes=1
  wires:
  Add/1 -> CAN send1/2(In2), Data Store Write/1  "dataBtx"
  Constant1/1 -> Add/2
  Data Store Read/1 -> Add/1
  Constant/1 -> CAN send1/1(In1)

== system HANcoder_E407_TTA_Chris/HANcoder STM32 Target - E407-STM32 algorithm/Enabled Subsystem/Trailer 2 ==
  In1 : Inport
  Enable : EnablePort
  Out1 : Outport
  wires:
  In1/1 -> Out1/1

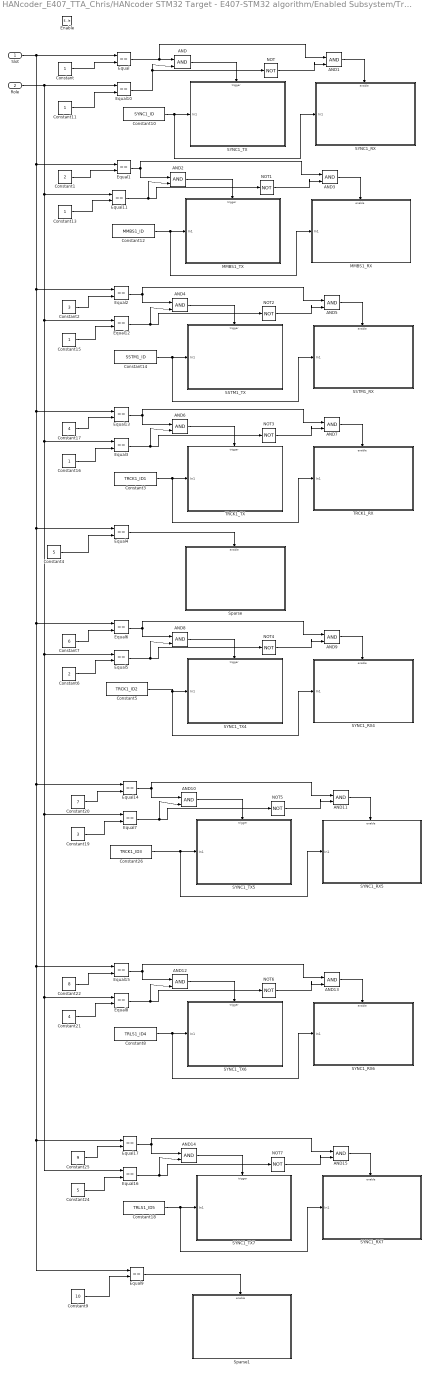
== system HANcoder_E407_TTA_Chris/HANcoder STM32 Target - E407-STM32 algorithm/Enabled Subsystem/Truck 1 ==
  Slot : Inport
  Role : Inport  Port=2
  Enable : EnablePort
  AND{,1..15} (16 alike) : Logic  IconShape=distinctive  AllPortsSameDT=off  OutDataTypeStr=boolean
  Constant{,11,13,15..16} (5 alike) : Constant
  Constant1 : Constant  Value=2
  Constant10 : Constant  Value=SYNC1_ID  OutDataTypeStr=uint32
  Constant12 : Constant  Value=MMBS1_ID  OutDataTypeStr=uint32
  Constant14 : Constant  Value=SSTM1_ID  OutDataTypeStr=uint32
  Constant17 : Constant  Value=4
  Constant18 : Constant  Value=TRLS1_ID5  OutDataTypeStr=uint32
  Constant19 : Constant  Value=3
  Constant2 : Constant  Value=3
  Constant20 : Constant  Value=7
  Constant21 : Constant  Value=4
  Constant22 : Constant  Value=8
  Constant24 : Constant  Value=5
  Constant25 : Constant  Value=9
  Constant26 : Constant  Value=TRCK1_ID3  OutDataTypeStr=uint32
  Constant3 : Constant  Value=TRCK1_ID1  OutDataTypeStr=uint32
  Constant4 : Constant  Value=5
  Constant5 : Constant  Value=TRCK1_ID2  OutDataTypeStr=uint32
  Constant6 : Constant  Value=2
  Constant7 : Constant  Value=6
  Constant8 : Constant  Value=TRLS1_ID4  OutDataTypeStr=uint32
  Constant9 : Constant  Value=10
  Equal{,1..17} (18 alike) : RelationalOperator  Operator===  OutDataTypeStr=boolean  RndMeth=Simplest  InputSameDT=off
  MMBS1_RX : Subsystem
  MMBS1_TX : Subsystem
  NOT{,1..7} (8 alike) : Logic  Operator=NOT  IconShape=distinctive  AllPortsSameDT=off  OutDataTypeStr=boolean
  SSTM1_RX : Subsystem
  SSTM1_TX : Subsystem
  SYNC1_RX : Subsystem
  SYNC1_RX4 : Subsystem
  SYNC1_RX5 : Subsystem
  SYNC1_RX6 : Subsystem
  SYNC1_RX7 : Subsystem
  SYNC1_TX : Subsystem
  SYNC1_TX4 : Subsystem
  SYNC1_TX5 : Subsystem
  SYNC1_TX6 : Subsystem
  SYNC1_TX7 : Subsystem
  Sparse : Subsystem
  Sparse1 : Subsystem
  TRCK1_RX : Subsystem
  TRCK1_TX : Subsystem
  wires:
  Constant/1 -> Equal/2
  Constant1/1 -> Equal1/2
  Constant2/1 -> Equal2/2
  Constant4/1 -> Equal4/2
  Equal4/1 -> Sparse/Enable
  Equal9/1 -> Sparse1/Enable
  Constant9/1 -> Equal9/2
  Constant10/1 -> SYNC1_RX/1(In1), SYNC1_TX/1(In1)
  AND/1 -> SYNC1_TX/Trigger
  Equal/1 -> AND1/1, AND/1
  AND1/1 -> SYNC1_RX/Enable
  Equal10/1 -> AND/2, NOT/1
  NOT/1 -> AND1/2
  Constant11/1 -> Equal10/2
  Equal1/1 -> AND3/1, AND2/1
  Constant12/1 -> MMBS1_RX/1(In1), MMBS1_TX/1(In1)
  NOT1/1 -> AND3/2
  Equal11/1 -> AND2/2, NOT1/1
  AND2/1 -> MMBS1_TX/Trigger
  AND3/1 -> MMBS1_RX/Enable
  Constant13/1 -> Equal11/2
  Equal12/1 -> AND4/2, NOT2/1
  NOT2/1 -> AND5/2
  AND4/1 -> SSTM1_TX/Trigger
  Constant14/1 -> SSTM1_RX/1(In1), SSTM1_TX/1(In1)
  AND5/1 -> SSTM1_RX/Enable
  Equal2/1 -> AND5/1, AND4/1
  Constant15/1 -> Equal12/2
  Constant16/1 -> Equal3/2
  Equal13/1 -> AND7/1, AND6/1
  Equal3/1 -> AND6/2, NOT3/1
  AND7/1 -> TRCK1_RX/Enable
  Constant3/1 -> TRCK1_RX/1(In1), TRCK1_TX/1(In1)
  AND6/1 -> TRCK1_TX/Trigger
  NOT3/1 -> AND7/2
  Constant17/1 -> Equal13/2
  Constant6/1 -> Equal5/2
  Equal6/1 -> AND9/1, AND8/1
  Equal5/1 -> AND8/2, NOT4/1
  AND9/1 -> SYNC1_RX4/Enable
  Constant5/1 -> SYNC1_RX4/1(In1), SYNC1_TX4/1(In1)
  AND8/1 -> SYNC1_TX4/Trigger
  NOT4/1 -> AND9/2
  Constant7/1 -> Equal6/2
  Constant19/1 -> Equal7/2
  Equal14/1 -> AND11/1, AND10/1
  Equal7/1 -> AND10/2, NOT5/1
  AND11/1 -> SYNC1_RX5/Enable
  Constant26/1 -> SYNC1_RX5/1(In1), SYNC1_TX5/1(In1)
  AND10/1 -> SYNC1_TX5/Trigger
  NOT5/1 -> AND11/2
  Constant20/1 -> Equal14/2
  Constant21/1 -> Equal8/2
  Equal15/1 -> AND13/1, AND12/1
  Equal8/1 -> AND12/2, NOT6/1
  AND13/1 -> SYNC1_RX6/Enable
  Constant8/1 -> SYNC1_RX6/1(In1), SYNC1_TX6/1(In1)
  AND12/1 -> SYNC1_TX6/Trigger
  NOT6/1 -> AND13/2
  Constant22/1 -> Equal15/2
  Constant24/1 -> Equal16/2
  Equal17/1 -> AND15/1, AND14/1
  Role/1 -> Equal16/1, Equal8/1, Equal7/1, Equal5/1, Equal3/1, Equal12/1, Equal11/1, Equal10/1
  Slot/1 -> Equal13/1, Equal6/1, Equal14/1, Equal15/1, Equal17/1, Equal9/1, Equal4/1, Equal2/1, Equal1/1, Equal/1
  Equal16/1 -> AND14/2, NOT7/1
  AND15/1 -> SYNC1_RX7/Enable
  Constant18/1 -> SYNC1_RX7/1(In1), SYNC1_TX7/1(In1)
  AND14/1 -> SYNC1_TX7/Trigger
  NOT7/1 -> AND15/2
  Constant25/1 -> Equal17/2

== system HANcoder_E407_TTA_Chris/HANcoder STM32 Target - E407-STM32 algorithm/Local Time generation/Enabled Subsystem ==
  Trigger : TriggerPort  VariantControl=(inherit)  PortDimensions=1
  Cast : DataTypeConversion  OutDataTypeStr=uint8  SaturateOnIntegerOverflow=off  RndMeth=Floor
  Constant : Constant  OutDataTypeStr=uint8
  Constant1 : Constant  Value=matrixRows
  Constant2 : Constant
  Constant3 : Constant  Value=0  OutDataTypeStr=uint16
  Data Store Read : DataStoreRead  DataStoreName=slot  IndexOptions=Index vector (dialog)  Indices=1  OutputSizes=1
  Data Store Read1 : DataStoreRead  DataStoreName=slot  IndexOptions=Index vector (dialog)  Indices=1  OutputSizes=1
  Data Store Write : DataStoreWrite  DataStoreName=slot  IndexOptions=Index vector (dialog)  Indices=1  OutputSizes=1
  Data Store Write1 : DataStoreWrite  DataStoreName=Local_Ticks  IndexOptions=Index vector (dialog)  Indices=1  OutputSizes=1
  Equal : RelationalOperator  Operator=<  OutDataTypeStr=boolean  RndMeth=Simplest  InputSameDT=off
  Plus : Sum  AccumDataTypeStr=uint8
  Switch : Switch  Criteria=u2 > Threshold  OutDataTypeStr=uint8  SaturateOnIntegerOverflow=off  InputSameDT=off
  Out1 : Outport
  wires:
  Data Store Read/1 -> Plus/1
  Constant/1 -> Plus/2
  Plus/1 -> Switch/1
  Switch/1 -> Out1/1, Data Store Write/1  "slotSelected"
  Equal/1 -> Switch/2
  Data Store Read1/1 -> Equal/1
  Constant1/1 -> Cast/1
  Constant2/1 -> Switch/3
  Constant3/1 -> Data Store Write1/1
  Cast/1 -> Equal/2

== system HANcoder_E407_TTA_Chris/HANcoder STM32 Target - E407-STM32 algorithm/Role assignment/Subsystem ==
  Trigger : TriggerPort  VariantControl=(inherit)  PortDimensions=1
  CAN send : Subsystem  Tag=HANcoder_TARGET_STM32_E407  AncestorBlock=HANcoder_STM32_Target/STM32-E407/CAN/CAN/CAN send  mask(CAN send){canBus=CAN 1, frameType=Standard (11 bit), inputNumber=1, dataType=uint8, byteOrder=on, tsamp=-1}
      mask prompts: canBus "CAN channel"; frameType "Identifier type"; inputNumber "Input ports"; dataType "Input datatype"; byteOrder "Byte order: Checked = MSB first, unchecked = LSB first."; tsamp "Sample time"
      mask help:
      | Function
      | ==========
      | Send a message on the CAN channel.
      |
      | Parameters
      | ==========
      | CAN channel:           The CAN channel to send the message on.
      | Identifier type:         normal or extended ID's
      | Input ports:              The amount of input ports
      | Input datatype:        The datatype of the input ports
      | Byte order:               Select MSB or LSB first
      | Sample time:            -1 or divisible by base sample time [seconds]
      |
      | Input
      | ==========
      | Port 1:                   CAN ID(uint32) in hexadecimal ie: hex2dec('0a')
      | Port 2..9                CAN message data
      mask init:
      | sfcn_can_send_mcb(canBus, frameType, inputNumber, dataType, byteOrder)
      settings: LibrarySourceBlock=HANcoder_STM32_Target/STM32-E407/CAN/CAN/CAN send  MoveFcn=drawLogos
      mask Help: web('sfcn_can_send.html');
      mask TypeOptions canBus: CAN 1 | CAN 2
      mask TypeOptions frameType: Standard (11 bit) | Extended (29 bit)
      mask TypeOptions dataType: int8 | uint8 | int16 | uint16 | int32 | uint32 | boolean
      mask Display:
      | fprintf('Send on\nCAN %x', canBus);
      | port_label('input', 1, 'ID');patch([65 71 71],[8 14 2],[1 0 0]);patch([73 73 79],[14 2 8],[0 0 0.35]);
  Constant : Constant  OutDataTypeStr=uint32
  Constant1 : Constant  Value=0  OutDataTypeStr=uint16
  Constant2 : Constant  Value=0  OutDataTypeStr=uint8
  Constant3 : Constant  Value=slotTime  OutDataTypeStr=uint8
  Data Store Read : DataStoreRead  DataStoreName=SlotTime  IndexOptions=Index vector (dialog)  Indices=1  OutputSizes=1
  Data Store Write : DataStoreWrite  DataStoreName=SlotTime  IndexOptions=Index vector (dialog)  Indices=1  OutputSizes=1
  Data Store Write1 : DataStoreWrite  DataStoreName=Local_Ticks  IndexOptions=Index vector (dialog)  Indices=1  OutputSizes=1
  Data Store Write2 : DataStoreWrite  DataStoreName=msgA_Count  IndexOptions=Index vector (dialog)  Indices=1  OutputSizes=1
  wires:
  Constant3/1 -> Data Store Write/1
  Constant/1 -> CAN send/1(In1)
  Data Store Read/1 -> CAN send/2(In2)
  Constant1/1 -> Data Store Write1/1
  Constant2/1 -> Data Store Write2/1

== system HANcoder_E407_TTA_Chris/HANcoder STM32 Target - E407-STM32 algorithm/Role assignment/Subsystem1 ==
  Enable : EnablePort
  CAN receive : Subsystem  Tag=HANcoder_TARGET_STM32_E407  AncestorBlock=HANcoder_STM32_Target/STM32-E407/CAN/CAN/CAN receive  mask(CAN receive){canBus=CAN 1, outputNumber=1, dataType=uint8, byteOrder=off, tsamp=-1}
      mask prompts: canBus "CAN channel"; outputNumber "Output ports"; dataType "Output datatype"; byteOrder "Byte order: Checked = MSB first, unchecked = LSB first."; tsamp "Sample time"
      mask help:
      | Function
      | ==========
      | Receive the newest message from the specified CAN channel.
      |
      | Parameters
      | ==========
      | CAN channel:             The CAN channel to send the message on.
      | Output ports:             The amount of output ports
      | Output datatype:       The datatype of the output ports
      | Byte order:                 Select MSB or LSB first
      | Sample time:              -1 or divisible by base sample time [seconds]
      |
      | Input
      | ==========
      | Port 1:                       CAN ID(uint32) in hexadecimal ie: hex2dec('0a')
      |
      | Output
      | ==========
      | Port 1:                       Checks for new message(int8)
      | Port 2..9                     Message data
      mask init:
      | sfcn_can_receive_mcb(canBus, outputNumber, dataType, byteOrder)
      settings: LibrarySourceBlock=HANcoder_STM32_Target/STM32-E407/CAN/CAN/CAN receive  MoveFcn=drawLogos
      mask Help: web('sfcn_can_receive.html');
      mask TypeOptions canBus: CAN 1 | CAN 2
      mask TypeOptions dataType: int8 | uint8 | int16 | uint16 | int32 | uint32 | boolean
      mask Display:
      | fprintf('Receive on\nCAN %x', canBus);
      | port_label('output', 1, 'new');
      | port_label('input', 1, 'ID');patch([75 81 81],[8 14 2],[1 0 0]);patch([83 83 89],[14 2 8],[0 0 0.35]);
  Cast : DataTypeConversion  OutDataTypeStr=boolean  SaturateOnIntegerOverflow=off  RndMeth=Floor
  Constant1 : Constant  OutDataTypeStr=uint32
  Data Store Write : DataStoreWrite  DataStoreName=SlotTime  IndexOptions=Index vector (dialog)  Indices=1  OutputSizes=1
  S-R Flip-Flop : simulink_extras/Flip Flops/S-R Flip-Flop  initial_condition=0
  Triggered Subsystem : Subsystem  TreatAsAtomicUnit=on
  Out1 : Outport
  wires:
  CAN receive/1(Out1) -> Cast/1
  Constant1/1 -> CAN receive/1(In1)
  CAN receive/2(Out2) -> Data Store Write/1
  S-R Flip-Flop/1 -> Out1/1
  Cast/1 -> Triggered Subsystem/Trigger, S-R Flip-Flop/1

== system HANcoder_E407_TTA_Chris/HANcoder STM32 Target - E407-STM32 algorithm/Communication/Role A Rx/CAN receive1 ==
  In1 : Inport
  Enabled Subsystem : Subsystem  TreatAsAtomicUnit=on
  S-Function : M-S-Function  FunctionName=sfcn_can_receive  Parameters=tsamp, canBus, outputNumber, dataType, byteOrder
  Term{3..9} (7 alike) : Terminator
  Out1 : Outport
  Out2 : Outport  Port=2
  wires:
  S-Function/9 -> Enabled Subsystem/8(In8)
  S-Function/4 -> Enabled Subsystem/3(In3)
  S-Function/5 -> Enabled Subsystem/4(In4)
  S-Function/8 -> Enabled Subsystem/7(In7)
  S-Function/7 -> Enabled Subsystem/6(In6)
  S-Function/6 -> Enabled Subsystem/5(In5)
  Enabled Subsystem/8(Out8) -> Term9/1
  Enabled Subsystem/7(Out7) -> Term8/1
  Enabled Subsystem/6(Out6) -> Term7/1
  Enabled Subsystem/5(Out5) -> Term6/1
  Enabled Subsystem/4(Out4) -> Term5/1
  Enabled Subsystem/3(Out3) -> Term4/1
  Enabled Subsystem/2(Out2) -> Term3/1
  Enabled Subsystem/1(Out1) -> Out2/1
  S-Function/3 -> Enabled Subsystem/2(In2)
  S-Function/2 -> Enabled Subsystem/1(In1)
  S-Function/1 -> Out1/1, Enabled Subsystem/Enable
  In1/1 -> S-Function/1

== system HANcoder_E407_TTA_Chris/HANcoder STM32 Target - E407-STM32 algorithm/Communication/Role A Tx/CAN send1 ==
  In1 : Inport
  In2 : Inport  Port=2
  Gnd{3..9} (7 alike) : Ground
  S-Function : M-S-Function  FunctionName=sfcn_can_send  Parameters=tsamp, canBus, frameType, inputNumber, dataType, byteOrder
  wires:
  In1/1 -> S-Function/1
  In2/1 -> S-Function/2
  Gnd3/1 -> S-Function/3
  Gnd4/1 -> S-Function/4
  Gnd5/1 -> S-Function/5
  Gnd6/1 -> S-Function/6
  Gnd7/1 -> S-Function/7
  Gnd8/1 -> S-Function/8
  Gnd9/1 -> S-Function/9

== system HANcoder_E407_TTA_Chris/HANcoder STM32 Target - E407-STM32 algorithm/Communication/Role B Rx/CAN receive1 ==
  In1 : Inport
  Enabled Subsystem : Subsystem  TreatAsAtomicUnit=on
  S-Function : M-S-Function  FunctionName=sfcn_can_receive  Parameters=tsamp, canBus, outputNumber, dataType, byteOrder
  Term{3..9} (7 alike) : Terminator
  Out1 : Outport
  Out2 : Outport  Port=2
  wires:
  S-Function/9 -> Enabled Subsystem/8(In8)
  S-Function/4 -> Enabled Subsystem/3(In3)
  S-Function/5 -> Enabled Subsystem/4(In4)
  S-Function/8 -> Enabled Subsystem/7(In7)
  S-Function/7 -> Enabled Subsystem/6(In6)
  S-Function/6 -> Enabled Subsystem/5(In5)
  Enabled Subsystem/8(Out8) -> Term9/1
  Enabled Subsystem/7(Out7) -> Term8/1
  Enabled Subsystem/6(Out6) -> Term7/1
  Enabled Subsystem/5(Out5) -> Term6/1
  Enabled Subsystem/4(Out4) -> Term5/1
  Enabled Subsystem/3(Out3) -> Term4/1
  Enabled Subsystem/2(Out2) -> Term3/1
  Enabled Subsystem/1(Out1) -> Out2/1
  S-Function/3 -> Enabled Subsystem/2(In2)
  S-Function/2 -> Enabled Subsystem/1(In1)
  S-Function/1 -> Out1/1, Enabled Subsystem/Enable
  In1/1 -> S-Function/1

== system HANcoder_E407_TTA_Chris/HANcoder STM32 Target - E407-STM32 algorithm/Communication/Role B Tx/CAN send1 ==
  In1 : Inport
  In2 : Inport  Port=2
  Gnd{3..9} (7 alike) : Ground
  S-Function : M-S-Function  FunctionName=sfcn_can_send  Parameters=tsamp, canBus, frameType, inputNumber, dataType, byteOrder
  wires:
  In1/1 -> S-Function/1
  In2/1 -> S-Function/2
  Gnd3/1 -> S-Function/3
  Gnd4/1 -> S-Function/4
  Gnd5/1 -> S-Function/5
  Gnd6/1 -> S-Function/6
  Gnd7/1 -> S-Function/7
  Gnd8/1 -> S-Function/8
  Gnd9/1 -> S-Function/9

== system HANcoder_E407_TTA_Chris/HANcoder STM32 Target - E407-STM32 algorithm/Enabled Subsystem/Truck 1/MMBS1_RX ==
  In1 : Inport
  Enable : EnablePort
  CAN receive1 : Subsystem  Tag=HANcoder_TARGET_STM32_E407  AncestorBlock=HANcoder_STM32_Target/STM32-E407/CAN/CAN/CAN receive  mask(CAN receive){canBus=CAN 1, outputNumber=1, dataType=uint8, byteOrder=off, tsamp=-1}
      mask prompts: canBus "CAN channel"; outputNumber "Output ports"; dataType "Output datatype"; byteOrder "Byte order: Checked = MSB first, unchecked = LSB first."; tsamp "Sample time"
      mask help:
      | Function
      | ==========
      | Receive the newest message from the specified CAN channel.
      |
      | Parameters
      | ==========
      | CAN channel:             The CAN channel to send the message on.
      | Output ports:             The amount of output ports
      | Output datatype:       The datatype of the output ports
      | Byte order:                 Select MSB or LSB first
      | Sample time:              -1 or divisible by base sample time [seconds]
      |
      | Input
      | ==========
      | Port 1:                       CAN ID(uint32) in hexadecimal ie: hex2dec('0a')
      |
      | Output
      | ==========
      | Port 1:                       Checks for new message(int8)
      | Port 2..9                     Message data
      mask init:
      | sfcn_can_receive_mcb(canBus, outputNumber, dataType, byteOrder)
      settings: LibrarySourceBlock=HANcoder_STM32_Target/STM32-E407/CAN/CAN/CAN receive  MoveFcn=drawLogos
      mask Help: web('sfcn_can_receive.html');
      mask TypeOptions canBus: CAN 1 | CAN 2
      mask TypeOptions dataType: int8 | uint8 | int16 | uint16 | int32 | uint32 | boolean
      mask Display:
      | fprintf('Receive on\nCAN %x', canBus);
      | port_label('output', 1, 'new');
      | port_label('input', 1, 'ID');patch([210 216 216],[8 14 2],[1 0 0]);patch([218 218 224],[14 2 8],[0 0 0.35]);
  Terminator : Terminator
  Terminator1 : Terminator
  wires:
  In1/1 -> CAN receive1/1(In1)
  CAN receive1/1(Out1) -> Terminator1/1
  CAN receive1/2(Out2) -> Terminator/1  "dataArx"

== system HANcoder_E407_TTA_Chris/HANcoder STM32 Target - E407-STM32 algorithm/Enabled Subsystem/Truck 1/MMBS1_TX ==
  In1 : Inport
  Trigger : TriggerPort  VariantControl=(inherit)  PortDimensions=1
  CAN send1 : Subsystem  Tag=HANcoder_TARGET_STM32_E407  AncestorBlock=HANcoder_STM32_Target/STM32-E407/CAN/CAN/CAN send  mask(CAN send){canBus=CAN 1, frameType=Standard (11 bit), inputNumber=1, dataType=uint8, byteOrder=on, tsamp=-1}
      mask prompts: canBus "CAN channel"; frameType "Identifier type"; inputNumber "Input ports"; dataType "Input datatype"; byteOrder "Byte order: Checked = MSB first, unchecked = LSB first."; tsamp "Sample time"
      mask help:
      | Function
      | ==========
      | Send a message on the CAN channel.
      |
      | Parameters
      | ==========
      | CAN channel:           The CAN channel to send the message on.
      | Identifier type:         normal or extended ID's
      | Input ports:              The amount of input ports
      | Input datatype:        The datatype of the input ports
      | Byte order:               Select MSB or LSB first
      | Sample time:            -1 or divisible by base sample time [seconds]
      |
      | Input
      | ==========
      | Port 1:                   CAN ID(uint32) in hexadecimal ie: hex2dec('0a')
      | Port 2..9                CAN message data
      mask init:
      | sfcn_can_send_mcb(canBus, frameType, inputNumber, dataType, byteOrder)
      settings: LibrarySourceBlock=HANcoder_STM32_Target/STM32-E407/CAN/CAN/CAN send  MoveFcn=drawLogos
      mask Help: web('sfcn_can_send.html');
      mask TypeOptions canBus: CAN 1 | CAN 2
      mask TypeOptions frameType: Standard (11 bit) | Extended (29 bit)
      mask TypeOptions dataType: int8 | uint8 | int16 | uint16 | int32 | uint32 | boolean
      mask Display:
      | fprintf('Send on\nCAN %x', canBus);
      | port_label('input', 1, 'ID');patch([200 206 206],[8 14 2],[1 0 0]);patch([208 208 214],[14 2 8],[0 0 0.35]);
  wires:
  In1/1 -> CAN send1/1(In1)
